simulink model "Test1_Mainor"  (R2023a)
settings: Solver=VariableStepAuto  StartTime=0.0  StopTime=5  FixedStep=1  RelTol=1e-3
settings Model: Creator=Hp  LastModifiedBy=Hp

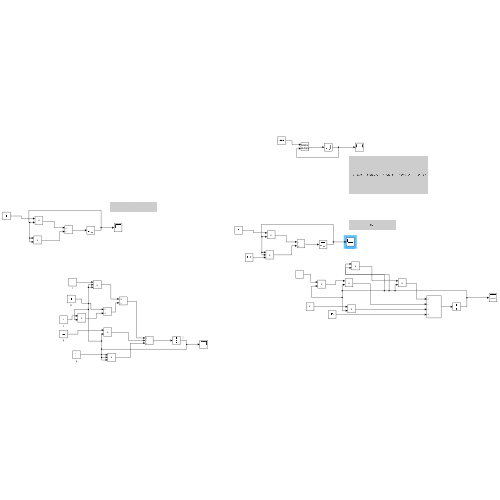
[thumbnail: Simulink's stored preview of the top-level diagram]
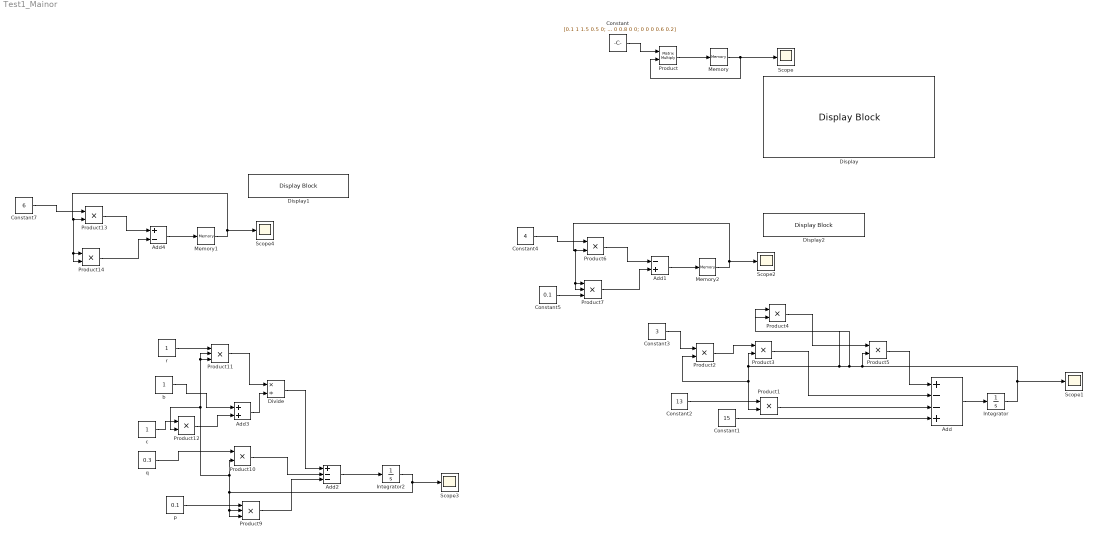
== system Test1_Mainor ==
  Add : Sum  Inputs=+--+
  Add1 : Sum  Inputs=-+
  Add2 : Sum  Inputs=+--
  Add3 : Sum
  Add4 : Sum  Inputs=+-
  Constant : Constant  Value=[0.1 1 1.5 0.5 0; 0.7 0 0 0 0; 0 0.8 0 0 0; 0 0 0.8 0 0; 0 0 0 0.6 0.2]
  Constant1 : Constant  Value=15
  Constant2 : Constant  Value=13
  Constant3 : Constant  Value=3
  Constant4 : Constant  Value=4
  Constant5 : Constant  Value=0.1
  Constant7 : Constant  Value=6
  Display : DisplayBlock  LabelPosition=Hide  Transparency=1
  Display1 : DisplayBlock  LabelPosition=Hide  Transparency=1
  Display2 : DisplayBlock  LabelPosition=Hide  Transparency=1
  Divide : Product  Inputs=*/
  Integrator : Integrator  InitialCondition=2
  Integrator2 : Integrator  InitialCondition=0.4
  Memory : Memory  InitialCondition=[100; 100; 300; 800; 100]
  Memory1 : Memory  InitialCondition=1
  Memory2 : Memory  InitialCondition=-2
  Product : Product  Multiplication=Matrix(*)
  Product{1..6,10,12..14} (10 alike) : Product
  Product11 : Product  Inputs=3
  Product7 : Product  Inputs=3
  Product9 : Product  Inputs=3
  Scope{,1..4} (5 alike) : Scope
  b : Constant
  c : Constant
  p : Constant  Value=0.1
  q : Constant  Value=0.3
  r : Constant
  wires:
  Constant/1 -> Product/1
  Product/1 -> Memory/1
  Memory/1 -> Scope/1, Product/2
  Add/1 -> Integrator/1
  Integrator/1 -> Scope1/1, Product5/2, Product4/1, Product4/2, Product2/2, Product1/2, Product3/2
  Constant3/1 -> Product2/1
  Product5/1 -> Add/1
  Constant2/1 -> Product1/1
  Product2/1 -> Product3/1
  Product1/1 -> Add/3
  Constant1/1 -> Add/4
  Product3/1 -> Add/2
  Product4/1 -> Product5/1
  Product11/1 -> Divide/1
  Add3/1 -> Divide/2
  Product12/1 -> Add3/2
  Product9/1 -> Add2/3
  Product10/1 -> Add2/2
  c/1 -> Product12/1
  Divide/1 -> Add2/1
  Integrator2/1 -> Scope3/1, Product12/2, Product11/3, Product11/2, Product10/2, Product9/3, Product9/2
  Add2/1 -> Integrator2/1
  p/1 -> Product9/1
  q/1 -> Product10/1
  b/1 -> Add3/1
  r/1 -> Product11/1
  Memory1/1 -> Scope4/1, Product14/2, Product14/1, Product13/2
  Add4/1 -> Memory1/1
  Constant7/1 -> Product13/1
  Product14/1 -> Add4/2
  Product13/1 -> Add4/1
  Memory2/1 -> Scope2/1, Product7/2, Product7/1, Product6/2
  Add1/1 -> Memory2/1
  Constant4/1 -> Product6/1
  Product7/1 -> Add1/2
  Product6/1 -> Add1/1
  Constant5/1 -> Product7/3
